simulink model "Mini4WD"  (R2016b)
settings: Solver=FixedStepAuto  StartTime=0.0  StopTime=10.0  RelTol=1e-3
undefined symbols (not defined in the file): SpeedFactorFromMyTuning, SpeedfactorFromWeight
settings Model: Creator=NEATdemo  LastModifiedBy=NEATdemo

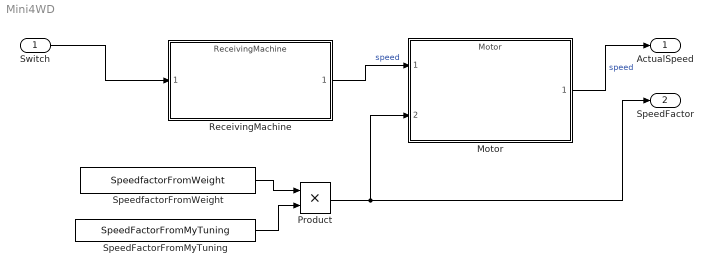
== system Mini4WD ==
  Switch : Inport
  Motor : ModelReference  ModelNameDialog=Motor  SimulationMode=Normal  ModelReferenceVersion=1.3
  Product : Product
  ReceivingMachine : ModelReference  ModelNameDialog=ReceivingMachine  SimulationMode=Normal  ModelReferenceVersion=1.11
  SpeedFactorFromMyTuning : Constant  Value=SpeedFactorFromMyTuning
  SpeedfactorFromWeight : Constant  Value=SpeedfactorFromWeight
  ActualSpeed : Outport
      settings: AttributesFormatString=speed
  SpeedFactor : Outport  Port=2
      settings: AttributesFormatString=SomethingFactor
  wires:
  ReceivingMachine/1 -> Motor/1  "speed"
  Switch/1 -> ReceivingMachine/1
  Motor/1 -> ActualSpeed/1  "speed"
  SpeedfactorFromWeight/1 -> Product/1
  SpeedFactorFromMyTuning/1 -> Product/2
  Product/1 -> SpeedFactor/1, Motor/2
